simulink subsystem "AeroPropRefFranc"  (R2024b)
settings: Solver=VariableStepAuto  StartTime=0.0  StopTime=10.0  RelTol=1e-3
undefined symbols (not defined in the file or in its folder): ess, Force_b, Fprop_r, geom, H_b, Hdot_b, Moment_b, mot, mot2, mot3, mot4, Mprop_r, propel, propel2, propel3, propel4, pxf_diagram_options, SimIn, SimPar, tc, tc2, tc3, tc4
libraries: simulink x8, slpidlib x4, starslibAxisTransformations x2, libAxisTransformations x2
(part 8 of 10)

== system AeroPropRefFranc/Propulsion and Aerodynamic Forces and Moments/S-Function/Battery Model/powerplant/mot4/plant/mot4_plant_map_Pelec_funTW_volt_in/non-zero division ==
  note: original idea from Phil Sharer - ANL
      | original formula: u[1]\(u[2]+eps)*(u[2]!=0)
      | changes done by Gerald ZINI (dgey) - ANL (05\02\2001)
  note: (u[2]==0) is true then returns 1, thus (u[2]+(u[2]==0)) is equal to 0+1=1
  note: if u[2] == 0, then output == 0:
  note: (u[2]!=0) is false then returns 0
  note: and finally, the expression is: (u[1] \ 1) * 0 = 0
  note: (u[2]==0) is false then returns 0, thus (u[2]+(u[2]==0)) is equal to u[2]+0=u[2]
  note: if u[2] != 0, then output == u[1]\u[2]:
  note: (u[2]!=0) is true then returns 1
  note: and finally, the expression is: (u[1] \ u[2]) * 1 = u[1] \ u[2]
  In1 : Inport
  In2 : Inport  Port=2
  Fcn : Fcn  Expr=u[1]/(u[2]+(u[2]==0))*(u[2]!=0)
  Mux : Mux  Inputs=2
  Out1 : Outport
  wires:
  Mux/1 -> Fcn/1
  In1/1 -> Mux/1
  Fcn/1 -> Out1/1
  In2/1 -> Mux/2

== system AeroPropRefFranc/Propulsion and Aerodynamic Forces and Moments/S-Function/Battery Model/powerplant/propel/plant/propel_plant_uas/Propeller Power ==
  propel_plant_CT_simu : Inport
  propel_plant_CP_simu : Inport  Port=2
  propel_plant_thrust_simu : Inport  Port=3
  propel_plant_rps_simu : Inport  Port=4
  eqnmotion_plant_linvel_simu : Inport  Port=5
  Dot Product : DotProduct  OutDataTypeStr=Inherit: Inherit via internal rule
  Fcn : Fcn  Expr=u(2) / u(1) * u(4) * u(3) * propel.plant.init.propD
  Mux : Mux
  Product : Product
  Sqrt : Sqrt
  propel_plant_pwr_in_simu : Outport  VectorParamsAs1DForOutWhenUnconnected=off
  propel_plant_pwr_out_simu : Outport  Port=2  VectorParamsAs1DForOutWhenUnconnected=off
  wires:
  propel_plant_CP_simu/1 -> Mux/2
  Fcn/1 -> propel_plant_pwr_in_simu/1  "propel_plant_pwr_in_simu"
  propel_plant_rps_simu/1 -> Mux/4
  propel_plant_thrust_simu/1 -> Product/1, Mux/3
  propel_plant_CT_simu/1 -> Mux/1
  Mux/1 -> Fcn/1
  Product/1 -> propel_plant_pwr_out_simu/1
  Sqrt/1 -> Product/2  "tas"
  eqnmotion_plant_linvel_simu/1 -> Dot Product/2, Dot Product/1
  Dot Product/1 -> Sqrt/1

== system AeroPropRefFranc/Propulsion and Aerodynamic Forces and Moments/S-Function/Battery Model/powerplant/propel/plant/propel_plant_uas/Propeller_CP ==
  propel_plant_rps_simu : Inport
  propel_plant_init_CP_CT_map : Subsystem  mask{x=propel.plant.init.CP_CT_map(:,1)/60, map=propel.plant.init.CP_CT_map(:,3)}
  propel_plant_CP_simu : Outport  VectorParamsAs1DForOutWhenUnconnected=off
  wires:
  propel_plant_rps_simu/1 -> propel_plant_init_CP_CT_map/1(input x)
  propel_plant_init_CP_CT_map/1(output) -> propel_plant_CP_simu/1

== system AeroPropRefFranc/Propulsion and Aerodynamic Forces and Moments/S-Function/Battery Model/powerplant/propel/plant/propel_plant_uas/Propeller_Torque ==
  note: I = Wprop*R^2/3g
      | General Aviation Aircraft Design pg 619
  env_plant_density_simu : Inport
  propel_plant_CP_simu : Inport  Port=2
  tc_plant_trq_out_simu : Inport  Port=3
  tc_plant_inertia_out_simu : Inport  Port=4
  " " : Gain  Gain=-1
  "2pi " : Gain  Gain=1/2/pi
  Demux : Demux  Outputs=2
  Fcn1 : Fcn  Expr=(u(1)/(2*pi)) *u(3)*(u(2)^2)*(propel.plant.init.propD^5)
  Integrator1 : Integrator  InitialCondition=propel.ctrl.init.rps
  Mux : Mux  Inputs=3
  Product : Product  Inputs=*/
  Prop Inertia : Constant  Value=propel.plant.init.Iprop
  Sum1 : Sum  Inputs=|+-
  Sum2 : Sum  Inputs=|++
  Terminator : Terminator
  propel_plant_rps_simu : Outport  VectorParamsAs1DForOutWhenUnconnected=off
  propel_plant_restq_simu : Outport  Port=2  VectorParamsAs1DForOutWhenUnconnected=off
  wires:
  Product/1 -> "2pi "/1
  Sum1/1 -> Product/1
  Sum2/1 -> Product/2
  tc_plant_inertia_out_simu/1 -> Sum2/2
  Prop Inertia/1 -> Sum2/1
  Fcn1/1 -> " "/1, Sum1/2  "propel_plant_restq_simu"
  tc_plant_trq_out_simu/1 -> Demux/1
  propel_plant_CP_simu/1 -> Mux/1  "prop_plant_CP_simu"
  env_plant_density_simu/1 -> Mux/3  "env_plant_density_simu"
  Integrator1/1 -> Mux/2, propel_plant_rps_simu/1  "propeller_plant_rps_simu"
  " "/1 -> propel_plant_restq_simu/1
  Mux/1 -> Fcn1/1
  "2pi "/1 -> Integrator1/1
  Demux/1 -> Sum1/1
  Demux/2 -> Terminator/1

== system AeroPropRefFranc/Propulsion and Aerodynamic Forces and Moments/S-Function/Battery Model/powerplant/propel/plant/propel_plant_uas/Thrust_Generated ==
  env_plant_density_simu : Inport
  propel_plant_speed_simu : Inport  Port=2
  Mux5 : Mux  Inputs=3
  RPS2T : Fcn  Expr=u(2) * u(3) * propel.plant.init.propD^4 * u(1)^2
  propel_plant_init_CP_CT_map : Subsystem  mask{x=propel.plant.init.CP_CT_map(:,1)/60, map=propel.plant.init.CP_CT_map(:,2)}
  propel_plant_thrust_simu : Outport  VectorParamsAs1DForOutWhenUnconnected=off
  propel_plant_CT_simu : Outport  Port=2  VectorParamsAs1DForOutWhenUnconnected=off
  wires:
  RPS2T/1 -> propel_plant_thrust_simu/1
  Mux5/1 -> RPS2T/1
  propel_plant_speed_simu/1 -> Mux5/1, propel_plant_init_CP_CT_map/1(input x)
  env_plant_density_simu/1 -> Mux5/3
  propel_plant_init_CP_CT_map/1(output) -> Mux5/2, propel_plant_CT_simu/1

== system AeroPropRefFranc/Propulsion and Aerodynamic Forces and Moments/S-Function/Battery Model/powerplant/propel/plant/propel_plant_uas/Total_Moment ==
  propel_plant_thrust_simu : Inport
  propel_plant_restq_simu : Inport  Port=2
  Gain : Gain  Gain=-propel.plant.init.rotationdir
  Gain1 : Gain  Gain=propel.plant.init.thrustdir
  Moment_due_to_eng_position : Subsystem
  Sum2 : Sum  Inputs=|+-  SaturateOnIntegerOverflow=on
  Sum4 : Sum  SaturateOnIntegerOverflow=on
  geom.init.CG : Constant  Value=geom.init.CG
  propel.plant.init.pos : Constant  Value=propel.plant.init.pos
  accmoment_plant_totmoment_simu : Outport  VectorParamsAs1DForOutWhenUnconnected=off
  wires:
  Moment_due_to_eng_position/1(X Prod) -> Sum4/1
  propel_plant_thrust_simu/1 -> Gain1/1
  geom.init.CG/1 -> Sum2/2
  propel.plant.init.pos/1 -> Sum2/1
  Sum4/1 -> accmoment_plant_totmoment_simu/1  "accmoment_plant_totmoment_simu"
  Sum2/1 -> Moment_due_to_eng_position/1(Vec 1)
  Gain/1 -> Sum4/2
  Gain1/1 -> Moment_due_to_eng_position/2(Vec 2)
  propel_plant_restq_simu/1 -> Gain/1

== system AeroPropRefFranc/Propulsion and Aerodynamic Forces and Moments/S-Function/Battery Model/powerplant/propel2/plant/propel2_plant_uas/Propeller Power ==
  propel_plant_CT_simu : Inport
  propel_plant_CP_simu : Inport  Port=2
  propel_plant_thrust_simu : Inport  Port=3
  propel_plant_rps_simu : Inport  Port=4
  eqnmotion_plant_linvel_simu : Inport  Port=5
  Dot Product : DotProduct  OutDataTypeStr=Inherit: Inherit via internal rule
  Fcn : Fcn  Expr=u(2) / u(1) * u(4) * u(3) * propel2.plant.init.propD
  Mux : Mux
  Product : Product
  Sqrt : Sqrt
  propel_plant_pwr_in_simu : Outport  VectorParamsAs1DForOutWhenUnconnected=off
  propel_plant_pwr_out_simu : Outport  Port=2  VectorParamsAs1DForOutWhenUnconnected=off
  wires:
  propel_plant_CP_simu/1 -> Mux/2
  Fcn/1 -> propel_plant_pwr_in_simu/1  "propel_plant_pwr_in_simu"
  propel_plant_rps_simu/1 -> Mux/4
  propel_plant_thrust_simu/1 -> Product/1, Mux/3
  propel_plant_CT_simu/1 -> Mux/1
  Mux/1 -> Fcn/1
  Product/1 -> propel_plant_pwr_out_simu/1
  Sqrt/1 -> Product/2  "tas"
  eqnmotion_plant_linvel_simu/1 -> Dot Product/2, Dot Product/1
  Dot Product/1 -> Sqrt/1

== system AeroPropRefFranc/Propulsion and Aerodynamic Forces and Moments/S-Function/Battery Model/powerplant/propel2/plant/propel2_plant_uas/Propeller_CP ==
  propel_plant_rps_simu : Inport
  propel_plant_init_CP_CT_map : Subsystem  mask{x=propel2.plant.init.CP_CT_map(:,1)/60, map=propel2.plant.init.CP_CT_map(:,3)}
  propel_plant_CP_simu : Outport  VectorParamsAs1DForOutWhenUnconnected=off
  wires:
  propel_plant_rps_simu/1 -> propel_plant_init_CP_CT_map/1(input x)
  propel_plant_init_CP_CT_map/1(output) -> propel_plant_CP_simu/1

== system AeroPropRefFranc/Propulsion and Aerodynamic Forces and Moments/S-Function/Battery Model/powerplant/propel2/plant/propel2_plant_uas/Propeller_Torque ==
  note: I = Wprop*R^2/3g
      | General Aviation Aircraft Design pg 619
  env_plant_density_simu : Inport
  propel_plant_CP_simu : Inport  Port=2
  tc_plant_trq_out_simu : Inport  Port=3
  tc_plant_inertia_out_simu : Inport  Port=4
  " " : Gain  Gain=-1
  "2pi " : Gain  Gain=1/2/pi
  Demux : Demux  Outputs=2
  Fcn1 : Fcn  Expr=(u(1)/(2*pi)) *u(3)*(u(2)^2)*(propel2.plant.init.propD^5)
  Integrator1 : Integrator  InitialCondition=propel2.ctrl.init.rps
  Mux : Mux  Inputs=3
  Product : Product  Inputs=*/
  Prop Inertia : Constant  Value=propel2.plant.init.Iprop
  Sum1 : Sum  Inputs=|+-
  Sum2 : Sum  Inputs=|++
  Terminator : Terminator
  propel_plant_rps_simu : Outport  VectorParamsAs1DForOutWhenUnconnected=off
  propel_plant_restq_simu : Outport  Port=2  VectorParamsAs1DForOutWhenUnconnected=off
  wires:
  Product/1 -> "2pi "/1
  Sum1/1 -> Product/1
  Sum2/1 -> Product/2
  tc_plant_inertia_out_simu/1 -> Sum2/2
  Prop Inertia/1 -> Sum2/1
  Fcn1/1 -> " "/1, Sum1/2  "propel_plant_restq_simu"
  tc_plant_trq_out_simu/1 -> Demux/1
  propel_plant_CP_simu/1 -> Mux/1  "prop_plant_CP_simu"
  env_plant_density_simu/1 -> Mux/3  "env_plant_density_simu"
  Integrator1/1 -> Mux/2, propel_plant_rps_simu/1  "propeller_plant_rps_simu"
  " "/1 -> propel_plant_restq_simu/1
  Mux/1 -> Fcn1/1
  "2pi "/1 -> Integrator1/1
  Demux/1 -> Sum1/1
  Demux/2 -> Terminator/1

== system AeroPropRefFranc/Propulsion and Aerodynamic Forces and Moments/S-Function/Battery Model/powerplant/propel2/plant/propel2_plant_uas/Thrust_Generated ==
  env_plant_density_simu : Inport
  propel_plant_speed_simu : Inport  Port=2
  Mux5 : Mux  Inputs=3
  RPS2T : Fcn  Expr=u(2) * u(3) * propel2.plant.init.propD^4 * u(1)^2
  propel_plant_init_CP_CT_map : Subsystem  mask{x=propel2.plant.init.CP_CT_map(:,1)/60, map=propel2.plant.init.CP_CT_map(:,2)}
  propel_plant_thrust_simu : Outport  VectorParamsAs1DForOutWhenUnconnected=off
  propel_plant_CT_simu : Outport  Port=2  VectorParamsAs1DForOutWhenUnconnected=off
  wires:
  RPS2T/1 -> propel_plant_thrust_simu/1
  Mux5/1 -> RPS2T/1
  propel_plant_speed_simu/1 -> Mux5/1, propel_plant_init_CP_CT_map/1(input x)
  env_plant_density_simu/1 -> Mux5/3
  propel_plant_init_CP_CT_map/1(output) -> Mux5/2, propel_plant_CT_simu/1

== system AeroPropRefFranc/Propulsion and Aerodynamic Forces and Moments/S-Function/Battery Model/powerplant/propel2/plant/propel2_plant_uas/Total_Moment ==
  propel_plant_thrust_simu : Inport
  propel_plant_restq_simu : Inport  Port=2
  Gain : Gain  Gain=-propel2.plant.init.rotationdir
  Gain1 : Gain  Gain=propel2.plant.init.thrustdir
  Moment_due_to_eng_position : Subsystem
  Sum2 : Sum  Inputs=|+-  SaturateOnIntegerOverflow=on
  Sum4 : Sum  SaturateOnIntegerOverflow=on
  geom.init.CG : Constant  Value=geom.init.CG
  propel.plant.init.pos : Constant  Value=propel2.plant.init.pos
  accmoment_plant_totmoment_simu : Outport  VectorParamsAs1DForOutWhenUnconnected=off
  wires:
  Moment_due_to_eng_position/1(X Prod) -> Sum4/1
  propel_plant_thrust_simu/1 -> Gain1/1
  geom.init.CG/1 -> Sum2/2
  propel.plant.init.pos/1 -> Sum2/1
  Sum4/1 -> accmoment_plant_totmoment_simu/1  "accmoment_plant_totmoment_simu"
  Sum2/1 -> Moment_due_to_eng_position/1(Vec 1)
  Gain/1 -> Sum4/2
  Gain1/1 -> Moment_due_to_eng_position/2(Vec 2)
  propel_plant_restq_simu/1 -> Gain/1

== system AeroPropRefFranc/Propulsion and Aerodynamic Forces and Moments/S-Function/Battery Model/powerplant/propel3/plant/propel3_plant_uas/Propeller Power ==
  propel_plant_CT_simu : Inport
  propel_plant_CP_simu : Inport  Port=2
  propel_plant_thrust_simu : Inport  Port=3
  propel_plant_rps_simu : Inport  Port=4
  eqnmotion_plant_linvel_simu : Inport  Port=5
  Dot Product : DotProduct  OutDataTypeStr=Inherit: Inherit via internal rule
  Fcn : Fcn  Expr=u(2) / u(1) * u(4) * u(3) * propel3.plant.init.propD
  Mux : Mux
  Product : Product
  Sqrt : Sqrt
  propel_plant_pwr_in_simu : Outport  VectorParamsAs1DForOutWhenUnconnected=off
  propel_plant_pwr_out_simu : Outport  Port=2  VectorParamsAs1DForOutWhenUnconnected=off
  wires:
  propel_plant_CP_simu/1 -> Mux/2
  Fcn/1 -> propel_plant_pwr_in_simu/1  "propel_plant_pwr_in_simu"
  propel_plant_rps_simu/1 -> Mux/4
  propel_plant_thrust_simu/1 -> Product/1, Mux/3
  propel_plant_CT_simu/1 -> Mux/1
  Mux/1 -> Fcn/1
  Product/1 -> propel_plant_pwr_out_simu/1
  Sqrt/1 -> Product/2  "tas"
  eqnmotion_plant_linvel_simu/1 -> Dot Product/2, Dot Product/1
  Dot Product/1 -> Sqrt/1

== system AeroPropRefFranc/Propulsion and Aerodynamic Forces and Moments/S-Function/Battery Model/powerplant/propel3/plant/propel3_plant_uas/Propeller_CP ==
  propel_plant_rps_simu : Inport
  propel_plant_init_CP_CT_map : Subsystem  mask{x=propel3.plant.init.CP_CT_map(:,1)/60, map=propel3.plant.init.CP_CT_map(:,3)}
  propel_plant_CP_simu : Outport  VectorParamsAs1DForOutWhenUnconnected=off
  wires:
  propel_plant_rps_simu/1 -> propel_plant_init_CP_CT_map/1(input x)
  propel_plant_init_CP_CT_map/1(output) -> propel_plant_CP_simu/1

== system AeroPropRefFranc/Propulsion and Aerodynamic Forces and Moments/S-Function/Battery Model/powerplant/propel3/plant/propel3_plant_uas/Propeller_Torque ==
  note: I = Wprop*R^2/3g
      | General Aviation Aircraft Design pg 619
  env_plant_density_simu : Inport
  propel_plant_CP_simu : Inport  Port=2
  tc_plant_trq_out_simu : Inport  Port=3
  tc_plant_inertia_out_simu : Inport  Port=4
  " " : Gain  Gain=-1
  "2pi " : Gain  Gain=1/2/pi
  Demux : Demux  Outputs=2
  Fcn1 : Fcn  Expr=(u(1)/(2*pi)) *u(3)*(u(2)^2)*(propel3.plant.init.propD^5)
  Integrator1 : Integrator  InitialCondition=propel3.ctrl.init.rps
  Mux : Mux  Inputs=3
  Product : Product  Inputs=*/
  Prop Inertia : Constant  Value=propel3.plant.init.Iprop
  Sum1 : Sum  Inputs=|+-
  Sum2 : Sum  Inputs=|++
  Terminator : Terminator
  propel_plant_rps_simu : Outport  VectorParamsAs1DForOutWhenUnconnected=off
  propel_plant_restq_simu : Outport  Port=2  VectorParamsAs1DForOutWhenUnconnected=off
  wires:
  Product/1 -> "2pi "/1
  Sum1/1 -> Product/1
  Sum2/1 -> Product/2
  tc_plant_inertia_out_simu/1 -> Sum2/2
  Prop Inertia/1 -> Sum2/1
  Fcn1/1 -> " "/1, Sum1/2  "propel_plant_restq_simu"
  tc_plant_trq_out_simu/1 -> Demux/1
  propel_plant_CP_simu/1 -> Mux/1  "prop_plant_CP_simu"
  env_plant_density_simu/1 -> Mux/3  "env_plant_density_simu"
  Integrator1/1 -> Mux/2, propel_plant_rps_simu/1  "propeller_plant_rps_simu"
  " "/1 -> propel_plant_restq_simu/1
  Mux/1 -> Fcn1/1
  "2pi "/1 -> Integrator1/1
  Demux/1 -> Sum1/1
  Demux/2 -> Terminator/1

== system AeroPropRefFranc/Propulsion and Aerodynamic Forces and Moments/S-Function/Battery Model/powerplant/propel3/plant/propel3_plant_uas/Thrust_Generated ==
  env_plant_density_simu : Inport
  propel_plant_speed_simu : Inport  Port=2
  Mux5 : Mux  Inputs=3
  RPS2T : Fcn  Expr=u(2) * u(3) * propel3.plant.init.propD^4 * u(1)^2
  propel_plant_init_CP_CT_map : Subsystem  mask{x=propel3.plant.init.CP_CT_map(:,1)/60, map=propel3.plant.init.CP_CT_map(:,2)}
  propel_plant_thrust_simu : Outport  VectorParamsAs1DForOutWhenUnconnected=off
  propel_plant_CT_simu : Outport  Port=2  VectorParamsAs1DForOutWhenUnconnected=off
  wires:
  RPS2T/1 -> propel_plant_thrust_simu/1
  Mux5/1 -> RPS2T/1
  propel_plant_speed_simu/1 -> Mux5/1, propel_plant_init_CP_CT_map/1(input x)
  env_plant_density_simu/1 -> Mux5/3
  propel_plant_init_CP_CT_map/1(output) -> Mux5/2, propel_plant_CT_simu/1

== system AeroPropRefFranc/Propulsion and Aerodynamic Forces and Moments/S-Function/Battery Model/powerplant/propel3/plant/propel3_plant_uas/Total_Moment ==
  propel_plant_thrust_simu : Inport
  propel_plant_restq_simu : Inport  Port=2
  Gain : Gain  Gain=-propel3.plant.init.rotationdir
  Gain1 : Gain  Gain=propel3.plant.init.thrustdir
  Moment_due_to_eng_position : Subsystem
  Sum2 : Sum  Inputs=|+-  SaturateOnIntegerOverflow=on
  Sum4 : Sum  SaturateOnIntegerOverflow=on
  geom.init.CG : Constant  Value=geom.init.CG
  propel.plant.init.pos : Constant  Value=propel3.plant.init.pos
  accmoment_plant_totmoment_simu : Outport  VectorParamsAs1DForOutWhenUnconnected=off
  wires:
  Moment_due_to_eng_position/1(X Prod) -> Sum4/1
  propel_plant_thrust_simu/1 -> Gain1/1
  geom.init.CG/1 -> Sum2/2
  propel.plant.init.pos/1 -> Sum2/1
  Sum4/1 -> accmoment_plant_totmoment_simu/1  "accmoment_plant_totmoment_simu"
  Sum2/1 -> Moment_due_to_eng_position/1(Vec 1)
  Gain/1 -> Sum4/2
  Gain1/1 -> Moment_due_to_eng_position/2(Vec 2)
  propel_plant_restq_simu/1 -> Gain/1

== system AeroPropRefFranc/Propulsion and Aerodynamic Forces and Moments/S-Function/Battery Model/powerplant/propel4/plant/propel4_plant_uas/Propeller Power ==
  propel_plant_CT_simu : Inport
  propel_plant_CP_simu : Inport  Port=2
  propel_plant_thrust_simu : Inport  Port=3
  propel_plant_rps_simu : Inport  Port=4
  eqnmotion_plant_linvel_simu : Inport  Port=5
  Dot Product : DotProduct  OutDataTypeStr=Inherit: Inherit via internal rule
  Fcn : Fcn  Expr=u(2) / u(1) * u(4) * u(3) * propel4.plant.init.propD
  Mux : Mux
  Product : Product
  Sqrt : Sqrt
  propel_plant_pwr_in_simu : Outport  VectorParamsAs1DForOutWhenUnconnected=off
  propel_plant_pwr_out_simu : Outport  Port=2  VectorParamsAs1DForOutWhenUnconnected=off
  wires:
  propel_plant_CP_simu/1 -> Mux/2
  Fcn/1 -> propel_plant_pwr_in_simu/1  "propel_plant_pwr_in_simu"
  propel_plant_rps_simu/1 -> Mux/4
  propel_plant_thrust_simu/1 -> Product/1, Mux/3
  propel_plant_CT_simu/1 -> Mux/1
  Mux/1 -> Fcn/1
  Product/1 -> propel_plant_pwr_out_simu/1
  Sqrt/1 -> Product/2  "tas"
  eqnmotion_plant_linvel_simu/1 -> Dot Product/2, Dot Product/1
  Dot Product/1 -> Sqrt/1

== system AeroPropRefFranc/Propulsion and Aerodynamic Forces and Moments/S-Function/Battery Model/powerplant/propel4/plant/propel4_plant_uas/Propeller_CP ==
  propel_plant_rps_simu : Inport
  propel_plant_init_CP_CT_map : Subsystem  mask{x=propel4.plant.init.CP_CT_map(:,1)/60, map=propel4.plant.init.CP_CT_map(:,3)}
  propel_plant_CP_simu : Outport  VectorParamsAs1DForOutWhenUnconnected=off
  wires:
  propel_plant_rps_simu/1 -> propel_plant_init_CP_CT_map/1(input x)
  propel_plant_init_CP_CT_map/1(output) -> propel_plant_CP_simu/1

== system AeroPropRefFranc/Propulsion and Aerodynamic Forces and Moments/S-Function/Battery Model/powerplant/propel4/plant/propel4_plant_uas/Propeller_Torque ==
  note: I = Wprop*R^2/3g
      | General Aviation Aircraft Design pg 619
  env_plant_density_simu : Inport
  propel_plant_CP_simu : Inport  Port=2
  tc_plant_trq_out_simu : Inport  Port=3
  tc_plant_inertia_out_simu : Inport  Port=4
  " " : Gain  Gain=-1
  "2pi " : Gain  Gain=1/2/pi
  Demux : Demux  Outputs=2
  Fcn1 : Fcn  Expr=(u(1)/(2*pi)) *u(3)*(u(2)^2)*(propel4.plant.init.propD^5)
  Integrator1 : Integrator  InitialCondition=propel4.ctrl.init.rps
  Mux : Mux  Inputs=3
  Product : Product  Inputs=*/
  Prop Inertia : Constant  Value=propel4.plant.init.Iprop
  Sum1 : Sum  Inputs=|+-
  Sum2 : Sum  Inputs=|++
  Terminator : Terminator
  propel_plant_rps_simu : Outport  VectorParamsAs1DForOutWhenUnconnected=off
  propel_plant_restq_simu : Outport  Port=2  VectorParamsAs1DForOutWhenUnconnected=off
  wires:
  Product/1 -> "2pi "/1
  Sum1/1 -> Product/1
  Sum2/1 -> Product/2
  tc_plant_inertia_out_simu/1 -> Sum2/2
  Prop Inertia/1 -> Sum2/1
  Fcn1/1 -> " "/1, Sum1/2  "propel_plant_restq_simu"
  tc_plant_trq_out_simu/1 -> Demux/1
  propel_plant_CP_simu/1 -> Mux/1  "prop_plant_CP_simu"
  env_plant_density_simu/1 -> Mux/3  "env_plant_density_simu"
  Integrator1/1 -> Mux/2, propel_plant_rps_simu/1  "propeller_plant_rps_simu"
  " "/1 -> propel_plant_restq_simu/1
  Mux/1 -> Fcn1/1
  "2pi "/1 -> Integrator1/1
  Demux/1 -> Sum1/1
  Demux/2 -> Terminator/1

== system AeroPropRefFranc/Propulsion and Aerodynamic Forces and Moments/S-Function/Battery Model/powerplant/propel4/plant/propel4_plant_uas/Thrust_Generated ==
  env_plant_density_simu : Inport
  propel_plant_speed_simu : Inport  Port=2
  Mux5 : Mux  Inputs=3
  RPS2T : Fcn  Expr=u(2) * u(3) * propel4.plant.init.propD^4 * u(1)^2
  propel_plant_init_CP_CT_map : Subsystem  mask{x=propel4.plant.init.CP_CT_map(:,1)/60, map=propel4.plant.init.CP_CT_map(:,2)}
  propel_plant_thrust_simu : Outport  VectorParamsAs1DForOutWhenUnconnected=off
  propel_plant_CT_simu : Outport  Port=2  VectorParamsAs1DForOutWhenUnconnected=off
  wires:
  RPS2T/1 -> propel_plant_thrust_simu/1
  Mux5/1 -> RPS2T/1
  propel_plant_speed_simu/1 -> Mux5/1, propel_plant_init_CP_CT_map/1(input x)
  env_plant_density_simu/1 -> Mux5/3
  propel_plant_init_CP_CT_map/1(output) -> Mux5/2, propel_plant_CT_simu/1

== system AeroPropRefFranc/Propulsion and Aerodynamic Forces and Moments/S-Function/Battery Model/powerplant/propel4/plant/propel4_plant_uas/Total_Moment ==
  propel_plant_thrust_simu : Inport
  propel_plant_restq_simu : Inport  Port=2
  Gain : Gain  Gain=-propel4.plant.init.rotationdir
  Gain1 : Gain  Gain=propel4.plant.init.thrustdir
  Moment_due_to_eng_position : Subsystem
  Sum2 : Sum  Inputs=|+-  SaturateOnIntegerOverflow=on
  Sum4 : Sum  SaturateOnIntegerOverflow=on
  geom.init.CG : Constant  Value=geom.init.CG
  propel.plant.init.pos : Constant  Value=propel4.plant.init.pos
  accmoment_plant_totmoment_simu : Outport  VectorParamsAs1DForOutWhenUnconnected=off
  wires:
  Moment_due_to_eng_position/1(X Prod) -> Sum4/1
  propel_plant_thrust_simu/1 -> Gain1/1
  geom.init.CG/1 -> Sum2/2
  propel.plant.init.pos/1 -> Sum2/1
  Sum4/1 -> accmoment_plant_totmoment_simu/1  "accmoment_plant_totmoment_simu"
  Sum2/1 -> Moment_due_to_eng_position/1(Vec 1)
  Gain/1 -> Sum4/2
  Gain1/1 -> Moment_due_to_eng_position/2(Vec 2)
  propel_plant_restq_simu/1 -> Gain/1

== system AeroPropRefFranc/Propulsion and Aerodynamic Forces and Moments/S-Function/Battery Model/powerplant/tc/plant/tc_plant_map_trqloss_funTW/Inertia calculation ==
  inertia in : Inport
  Sum3 : Sum  Inputs=|++  InputSameDT=on  SaturateOnIntegerOverflow=on  OutDataTypeStr=Inherit: Same as first input
  tc inertia : Constant  Value=tc.plant.init.inertia
  tc.plant.init.ratio : Gain  Gain=tc.plant.init.ratio
  "tc.plant.init.ratio " : Gain  Gain=tc.plant.init.ratio
  inertia out : Outport
  wires:
  Sum3/1 -> inertia out/1
  tc inertia/1 -> Sum3/2
  tc.plant.init.ratio/1 -> Sum3/1
  inertia in/1 -> "tc.plant.init.ratio "/1
  "tc.plant.init.ratio "/1 -> tc.plant.init.ratio/1

== system AeroPropRefFranc/Propulsion and Aerodynamic Forces and Moments/S-Function/Battery Model/powerplant/tc/plant/tc_plant_map_trqloss_funTW/Speed calculation ==
  spd out : Inport
  tc.plant.init.ratio : Gain  Gain=tc.plant.init.ratio
  spd in : Outport
  wires:
  tc.plant.init.ratio/1 -> spd in/1
  spd out/1 -> tc.plant.init.ratio/1

== system AeroPropRefFranc/Propulsion and Aerodynamic Forces and Moments/S-Function/Battery Model/powerplant/tc/plant/tc_plant_map_trqloss_funTW/Torque calculation ==
  spd in : Inport
  trq in : Inport  Port=2
  Abs : Abs
  Abs1 : Abs
  Blending (state dependent) : Subsystem  mask(State dependent blending){xl=-tc.plant.init.spd_thresh, yl=-1, xc=0, yc=0, xr=tc.plant.init.spd_thresh, yr=1}
      mask prompts: xl "Left point (x):"; yl "Left point (y):"; xc "Center point (x):"; yc "Center point (y):"; xr "Right point (x):"; yr "Right point (y):"
      mask help: This block implements state dependent smoothing/blending. IMPORTANT: See help menu.
      mask Help: The output equals the product of the first input and a "hat" function defined by the three points specified in the dialog box.  The second input forms the argument to the hat function.\n\nIMPORTANT: A divide by zero error will result if first coordinates of the three points specified for the hat function are NOT distinct.
      mask Display: plot([-1 1 3 6 8], [1.5 1.5 0.5 4.0 4.0])
  Sum2 : Sum  Inputs=|+-  InputSameDT=on  SaturateOnIntegerOverflow=on  OutDataTypeStr=Inherit: Same as first input
  tc.plant.init.ratio : Gain  Gain=tc.plant.init.ratio
  trq losses : Subsystem  mask(Lookup Table (2-D)){x=tc.plant.init.trq_loss.idx1_trq, y=tc.plant.init.trq_loss.idx2_spd, t=tc.plant.init.trq_loss.map}
      mask prompts: x "Row:"; y "Column:"; t "Table:"
      mask help: Performs 2-D linear interpolation of input values using the specified input/output table. Extrapolation is performed outside the table boundaries.
      mask init:
      | [r,c]=size(t);
      | xt=reshape(x,prod(size(x)),1);
      | xi=xt(:,ones(1,c));
      | minx=min(x); maxx=max(x);
      | mint=min(min(t)); maxt=max(max(t));
      mask Display: plot(xi,t,[minx maxx],[mint mint],[minx minx],[mint maxt])
  trq out : Outport
  wires:
  Abs/1 -> trq losses/1(Rows)
  Abs1/1 -> trq losses/2(Cols)
  trq losses/1(Out1) -> Blending (state dependent)/1(Input)
  Blending (state dependent)/1(Output) -> Sum2/2
  spd in/1 -> Abs1/1, Blending (state dependent)/2(Control (state))
  trq in/1 -> Abs/1, Sum2/1
  Sum2/1 -> tc.plant.init.ratio/1
  tc.plant.init.ratio/1 -> trq out/1

== system AeroPropRefFranc/Propulsion and Aerodynamic Forces and Moments/S-Function/Battery Model/powerplant/tc2/plant/tc2_plant_map_trqloss_funTW/Inertia calculation ==
  inertia in : Inport
  Sum3 : Sum  Inputs=|++  InputSameDT=on  SaturateOnIntegerOverflow=on  OutDataTypeStr=Inherit: Same as first input
  tc inertia : Constant  Value=tc2.plant.init.inertia
  tc.plant.init.ratio : Gain  Gain=tc2.plant.init.ratio
  "tc.plant.init.ratio " : Gain  Gain=tc2.plant.init.ratio
  inertia out : Outport
  wires:
  Sum3/1 -> inertia out/1
  tc inertia/1 -> Sum3/2
  tc.plant.init.ratio/1 -> Sum3/1
  inertia in/1 -> "tc.plant.init.ratio "/1
  "tc.plant.init.ratio "/1 -> tc.plant.init.ratio/1

== system AeroPropRefFranc/Propulsion and Aerodynamic Forces and Moments/S-Function/Battery Model/powerplant/tc2/plant/tc2_plant_map_trqloss_funTW/Speed calculation ==
  spd out : Inport
  tc.plant.init.ratio : Gain  Gain=tc2.plant.init.ratio
  spd in : Outport
  wires:
  tc.plant.init.ratio/1 -> spd in/1
  spd out/1 -> tc.plant.init.ratio/1

== system AeroPropRefFranc/Propulsion and Aerodynamic Forces and Moments/S-Function/Battery Model/powerplant/tc2/plant/tc2_plant_map_trqloss_funTW/Torque calculation ==
  spd in : Inport
  trq in : Inport  Port=2
  Abs : Abs
  Abs1 : Abs
  Blending (state dependent) : Subsystem  mask(State dependent blending){xl=-tc2.plant.init.spd_thresh, yl=-1, xc=0, yc=0, xr=tc2.plant.init.spd_thresh, yr=1}
      mask prompts: xl "Left point (x):"; yl "Left point (y):"; xc "Center point (x):"; yc "Center point (y):"; xr "Right point (x):"; yr "Right point (y):"
      mask help: This block implements state dependent smoothing/blending. IMPORTANT: See help menu.
      mask Help: The output equals the product of the first input and a "hat" function defined by the three points specified in the dialog box.  The second input forms the argument to the hat function.\n\nIMPORTANT: A divide by zero error will result if first coordinates of the three points specified for the hat function are NOT distinct.
      mask Display: plot([-1 1 3 6 8], [1.5 1.5 0.5 4.0 4.0])
  Sum2 : Sum  Inputs=|+-  InputSameDT=on  SaturateOnIntegerOverflow=on  OutDataTypeStr=Inherit: Same as first input
  tc.plant.init.ratio : Gain  Gain=tc2.plant.init.ratio
  trq losses : Subsystem  mask(Lookup Table (2-D)){x=tc2.plant.init.trq_loss.idx1_trq, y=tc2.plant.init.trq_loss.idx2_spd, t=tc2.plant.init.trq_loss.map}
      mask prompts: x "Row:"; y "Column:"; t "Table:"
      mask help: Performs 2-D linear interpolation of input values using the specified input/output table. Extrapolation is performed outside the table boundaries.
      mask init:
      | [r,c]=size(t);
      | xt=reshape(x,prod(size(x)),1);
      | xi=xt(:,ones(1,c));
      | minx=min(x); maxx=max(x);
      | mint=min(min(t)); maxt=max(max(t));
      mask Display: plot(xi,t,[minx maxx],[mint mint],[minx minx],[mint maxt])
  trq out : Outport
  wires:
  Abs/1 -> trq losses/1(Rows)
  Abs1/1 -> trq losses/2(Cols)
  trq losses/1(Out1) -> Blending (state dependent)/1(Input)
  Blending (state dependent)/1(Output) -> Sum2/2
  spd in/1 -> Abs1/1, Blending (state dependent)/2(Control (state))
  trq in/1 -> Abs/1, Sum2/1
  Sum2/1 -> tc.plant.init.ratio/1
  tc.plant.init.ratio/1 -> trq out/1

== system AeroPropRefFranc/Propulsion and Aerodynamic Forces and Moments/S-Function/Battery Model/powerplant/tc3/plant/tc3_plant_map_trqloss_funTW/Inertia calculation ==
  inertia in : Inport
  Sum3 : Sum  Inputs=|++  InputSameDT=on  SaturateOnIntegerOverflow=on  OutDataTypeStr=Inherit: Same as first input
  tc inertia : Constant  Value=tc3.plant.init.inertia
  tc.plant.init.ratio : Gain  Gain=tc3.plant.init.ratio
  "tc.plant.init.ratio " : Gain  Gain=tc3.plant.init.ratio
  inertia out : Outport
  wires:
  Sum3/1 -> inertia out/1
  tc inertia/1 -> Sum3/2
  tc.plant.init.ratio/1 -> Sum3/1
  inertia in/1 -> "tc.plant.init.ratio "/1
  "tc.plant.init.ratio "/1 -> tc.plant.init.ratio/1

== system AeroPropRefFranc/Propulsion and Aerodynamic Forces and Moments/S-Function/Battery Model/powerplant/tc3/plant/tc3_plant_map_trqloss_funTW/Speed calculation ==
  spd out : Inport
  tc.plant.init.ratio : Gain  Gain=tc3.plant.init.ratio
  spd in : Outport
  wires:
  tc.plant.init.ratio/1 -> spd in/1
  spd out/1 -> tc.plant.init.ratio/1

== system AeroPropRefFranc/Propulsion and Aerodynamic Forces and Moments/S-Function/Battery Model/powerplant/tc3/plant/tc3_plant_map_trqloss_funTW/Torque calculation ==
  spd in : Inport
  trq in : Inport  Port=2
  Abs : Abs
  Abs1 : Abs
  Blending (state dependent) : Subsystem  mask(State dependent blending){xl=-tc3.plant.init.spd_thresh, yl=-1, xc=0, yc=0, xr=tc3.plant.init.spd_thresh, yr=1}
      mask prompts: xl "Left point (x):"; yl "Left point (y):"; xc "Center point (x):"; yc "Center point (y):"; xr "Right point (x):"; yr "Right point (y):"
      mask help: This block implements state dependent smoothing/blending. IMPORTANT: See help menu.
      mask Help: The output equals the product of the first input and a "hat" function defined by the three points specified in the dialog box.  The second input forms the argument to the hat function.\n\nIMPORTANT: A divide by zero error will result if first coordinates of the three points specified for the hat function are NOT distinct.
      mask Display: plot([-1 1 3 6 8], [1.5 1.5 0.5 4.0 4.0])
  Sum2 : Sum  Inputs=|+-  InputSameDT=on  SaturateOnIntegerOverflow=on  OutDataTypeStr=Inherit: Same as first input
  tc.plant.init.ratio : Gain  Gain=tc3.plant.init.ratio
  trq losses : Subsystem  mask(Lookup Table (2-D)){x=tc3.plant.init.trq_loss.idx1_trq, y=tc3.plant.init.trq_loss.idx2_spd, t=tc3.plant.init.trq_loss.map}
      mask prompts: x "Row:"; y "Column:"; t "Table:"
      mask help: Performs 2-D linear interpolation of input values using the specified input/output table. Extrapolation is performed outside the table boundaries.
      mask init:
      | [r,c]=size(t);
      | xt=reshape(x,prod(size(x)),1);
      | xi=xt(:,ones(1,c));
      | minx=min(x); maxx=max(x);
      | mint=min(min(t)); maxt=max(max(t));
      mask Display: plot(xi,t,[minx maxx],[mint mint],[minx minx],[mint maxt])
  trq out : Outport
  wires:
  Abs/1 -> trq losses/1(Rows)
  Abs1/1 -> trq losses/2(Cols)
  trq losses/1(Out1) -> Blending (state dependent)/1(Input)
  Blending (state dependent)/1(Output) -> Sum2/2
  spd in/1 -> Abs1/1, Blending (state dependent)/2(Control (state))
  trq in/1 -> Abs/1, Sum2/1
  Sum2/1 -> tc.plant.init.ratio/1
  tc.plant.init.ratio/1 -> trq out/1

== system AeroPropRefFranc/Propulsion and Aerodynamic Forces and Moments/S-Function/Battery Model/powerplant/tc4/plant/tc4_plant_map_trqloss_funTW/Inertia calculation ==
  inertia in : Inport
  Sum3 : Sum  Inputs=|++  InputSameDT=on  SaturateOnIntegerOverflow=on  OutDataTypeStr=Inherit: Same as first input
  tc inertia : Constant  Value=tc4.plant.init.inertia
  tc.plant.init.ratio : Gain  Gain=tc4.plant.init.ratio
  "tc.plant.init.ratio " : Gain  Gain=tc4.plant.init.ratio
  inertia out : Outport
  wires:
  Sum3/1 -> inertia out/1
  tc inertia/1 -> Sum3/2
  tc.plant.init.ratio/1 -> Sum3/1
  inertia in/1 -> "tc.plant.init.ratio "/1
  "tc.plant.init.ratio "/1 -> tc.plant.init.ratio/1

== system AeroPropRefFranc/Propulsion and Aerodynamic Forces and Moments/S-Function/Battery Model/powerplant/tc4/plant/tc4_plant_map_trqloss_funTW/Speed calculation ==
  spd out : Inport
  tc.plant.init.ratio : Gain  Gain=tc4.plant.init.ratio
  spd in : Outport
  wires:
  tc.plant.init.ratio/1 -> spd in/1
  spd out/1 -> tc.plant.init.ratio/1

== system AeroPropRefFranc/Propulsion and Aerodynamic Forces and Moments/S-Function/Battery Model/powerplant/tc4/plant/tc4_plant_map_trqloss_funTW/Torque calculation ==
  spd in : Inport
  trq in : Inport  Port=2
  Abs : Abs
  Abs1 : Abs
  Blending (state dependent) : Subsystem  mask(State dependent blending){xl=-tc4.plant.init.spd_thresh, yl=-1, xc=0, yc=0, xr=tc4.plant.init.spd_thresh, yr=1}
      mask prompts: xl "Left point (x):"; yl "Left point (y):"; xc "Center point (x):"; yc "Center point (y):"; xr "Right point (x):"; yr "Right point (y):"
      mask help: This block implements state dependent smoothing/blending. IMPORTANT: See help menu.
      mask Help: The output equals the product of the first input and a "hat" function defined by the three points specified in the dialog box.  The second input forms the argument to the hat function.\n\nIMPORTANT: A divide by zero error will result if first coordinates of the three points specified for the hat function are NOT distinct.
      mask Display: plot([-1 1 3 6 8], [1.5 1.5 0.5 4.0 4.0])
  Sum2 : Sum  Inputs=|+-  InputSameDT=on  SaturateOnIntegerOverflow=on  OutDataTypeStr=Inherit: Same as first input
  tc.plant.init.ratio : Gain  Gain=tc4.plant.init.ratio
  trq losses : Subsystem  mask(Lookup Table (2-D)){x=tc4.plant.init.trq_loss.idx1_trq, y=tc4.plant.init.trq_loss.idx2_spd, t=tc4.plant.init.trq_loss.map}
      mask prompts: x "Row:"; y "Column:"; t "Table:"
      mask help: Performs 2-D linear interpolation of input values using the specified input/output table. Extrapolation is performed outside the table boundaries.
      mask init:
      | [r,c]=size(t);
      | xt=reshape(x,prod(size(x)),1);
      | xi=xt(:,ones(1,c));
      | minx=min(x); maxx=max(x);
      | mint=min(min(t)); maxt=max(max(t));
      mask Display: plot(xi,t,[minx maxx],[mint mint],[minx minx],[mint maxt])
  trq out : Outport
  wires:
  Abs/1 -> trq losses/1(Rows)
  Abs1/1 -> trq losses/2(Cols)
  trq losses/1(Out1) -> Blending (state dependent)/1(Input)
  Blending (state dependent)/1(Output) -> Sum2/2
  spd in/1 -> Abs1/1, Blending (state dependent)/2(Control (state))
  trq in/1 -> Abs/1, Sum2/1
  Sum2/1 -> tc.plant.init.ratio/1
  tc.plant.init.ratio/1 -> trq out/1

== system AeroPropRefFranc/Propulsion and Aerodynamic Forces and Moments/S-Function/Battery Model/ess (battery)/ctrl/ess_ctrl_pngv_map_anl_PI_cstr/PI controller for maximal charge power and current1/PI Ratio Calculator (curr) /non-zero division1 ==
  note: and finally, the expression is: (u[1] \ u[2]) * 1 = u[1] \ u[2]
  note: (u[2]!=0) is true then returns 1
  note: if u[2] != 0, then output == u[1]\u[2]:
  note: (u[2]==0) is false then returns 0, thus (u[2]+(u[2]==0)) is equal to u[2]+0=u[2]
  note: and finally, the expression is: (u[1] \ 1) * 0 = 0
  note: (u[2]!=0) is false then returns 0
  note: if u[2] == 0, then output == 0:
  note: (u[2]==0) is true then returns 1, thus (u[2]+(u[2]==0)) is equal to 0+1=1
  note: original idea from Phil Sharer - ANL
      | original formula: u[1]\(u[2]+eps)*(u[2]!=0)
      | changes done by Gerald ZINI (dgey) - ANL (05\02\2001)
  In1 : Inport
  In2 : Inport  Port=2
  Fcn : Fcn  Expr=u[1]/(u[2]+(u[2]==0))*(u[2]!=0)
  Mux : Mux  Inputs=2
  Out1 : Outport
  wires:
  In2/1 -> Mux/2
  Fcn/1 -> Out1/1
  In1/1 -> Mux/1
  Mux/1 -> Fcn/1

== system AeroPropRefFranc/Propulsion and Aerodynamic Forces and Moments/S-Function/Battery Model/ess (battery)/ctrl/ess_ctrl_pngv_map_anl_PI_cstr/PI controller for maximal charge power and current1/PI Ratio Calculator (curr) 1/non-zero division1 ==
  note: and finally, the expression is: (u[1] \ u[2]) * 1 = u[1] \ u[2]
  note: (u[2]!=0) is true then returns 1
  note: if u[2] != 0, then output == u[1]\u[2]:
  note: (u[2]==0) is false then returns 0, thus (u[2]+(u[2]==0)) is equal to u[2]+0=u[2]
  note: and finally, the expression is: (u[1] \ 1) * 0 = 0
  note: (u[2]!=0) is false then returns 0
  note: if u[2] == 0, then output == 0:
  note: (u[2]==0) is true then returns 1, thus (u[2]+(u[2]==0)) is equal to 0+1=1
  note: original idea from Phil Sharer - ANL
      | original formula: u[1]\(u[2]+eps)*(u[2]!=0)
      | changes done by Gerald ZINI (dgey) - ANL (05\02\2001)
  In1 : Inport
  In2 : Inport  Port=2
  Fcn : Fcn  Expr=u[1]/(u[2]+(u[2]==0))*(u[2]!=0)
  Mux : Mux  Inputs=2
  Out1 : Outport
  wires:
  In2/1 -> Mux/2
  Fcn/1 -> Out1/1
  In1/1 -> Mux/1
  Mux/1 -> Fcn/1

== system AeroPropRefFranc/Propulsion and Aerodynamic Forces and Moments/S-Function/Battery Model/ess (battery)/ctrl/ess_ctrl_pngv_map_anl_PI_cstr/PI controller for maximal discharge power and current1/PI Ratio Calculator (curr) /non-zero division1 ==
  note: original idea from Phil Sharer - ANL
      | original formula: u[1]\(u[2]+eps)*(u[2]!=0)
      | changes done by Gerald ZINI (dgey) - ANL (05\02\2001)
  note: (u[2]==0) is true then returns 1, thus (u[2]+(u[2]==0)) is equal to 0+1=1
  note: if u[2] == 0, then output == 0:
  note: (u[2]!=0) is false then returns 0
  note: and finally, the expression is: (u[1] \ 1) * 0 = 0
  note: (u[2]==0) is false then returns 0, thus (u[2]+(u[2]==0)) is equal to u[2]+0=u[2]
  note: if u[2] != 0, then output == u[1]\u[2]:
  note: (u[2]!=0) is true then returns 1
  note: and finally, the expression is: (u[1] \ u[2]) * 1 = u[1] \ u[2]
  In1 : Inport
  In2 : Inport  Port=2
  Fcn : Fcn  Expr=u[1]/(u[2]+(u[2]==0))*(u[2]!=0)
  Mux : Mux  Inputs=2
  Out1 : Outport
  wires:
  Mux/1 -> Fcn/1
  In1/1 -> Mux/1
  Fcn/1 -> Out1/1
  In2/1 -> Mux/2

== system AeroPropRefFranc/Propulsion and Aerodynamic Forces and Moments/S-Function/Battery Model/ess (battery)/ctrl/ess_ctrl_pngv_map_anl_PI_cstr/PI controller for maximal discharge power and current1/PI Ratio Calculator (curr) 1/non-zero division1 ==
  note: and finally, the expression is: (u[1] \ u[2]) * 1 = u[1] \ u[2]
  note: (u[2]!=0) is true then returns 1
  note: if u[2] != 0, then output == u[1]\u[2]:
  note: (u[2]==0) is false then returns 0, thus (u[2]+(u[2]==0)) is equal to u[2]+0=u[2]
  note: and finally, the expression is: (u[1] \ 1) * 0 = 0
  note: (u[2]!=0) is false then returns 0
  note: if u[2] == 0, then output == 0:
  note: (u[2]==0) is true then returns 1, thus (u[2]+(u[2]==0)) is equal to 0+1=1
  note: original idea from Phil Sharer - ANL
      | original formula: u[1]\(u[2]+eps)*(u[2]!=0)
      | changes done by Gerald ZINI (dgey) - ANL (05\02\2001)
  In1 : Inport
  In2 : Inport  Port=2
  Fcn : Fcn  Expr=u[1]/(u[2]+(u[2]==0))*(u[2]!=0)
  Mux : Mux  Inputs=2
  Out1 : Outport
  wires:
  In2/1 -> Mux/2
  Fcn/1 -> Out1/1
  In1/1 -> Mux/1
  Mux/1 -> Fcn/1

== system AeroPropRefFranc/Propulsion and Aerodynamic Forces and Moments/S-Function/Battery Model/powerplant/ess (battery)/ctrl/ess_ctrl_pngv_map_anl_PI_cstr/PI controller for maximal charge power and current1/PI Ratio Calculator (curr)  ==
  note: %deviation
  ess curr : Inport
  curr max cont : Inport  Port=2
  Add1 : Sum  Inputs=-+
  Integrator1 : Integrator  InitialCondition=ess.plant.init.ul_curr_chg  LimitOutput=on  UpperSaturationLimit=ess.plant.init.ul_curr_chg  LowerSaturationLimit=ess.plant.init.ll_curr_chg
  Ki_curr : Gain  Gain=ess.plant.init.Ki_curr_chg  SaturateOnIntegerOverflow=on  OutDataTypeStr=Inherit: Same as input  ParamDataTypeStr=Inherit: Same as input
  Saturation1 : Saturate  UpperLimit=1  LowerLimit=0
  non-zero division1 : Subsystem
      mask Display: disp('divider')
  Current ratio : Outport
  wires:
  curr max cont/1 -> non-zero division1/2(In2), Add1/2
  Saturation1/1 -> Current ratio/1
  ess curr/1 -> Add1/1
  Integrator1/1 -> Saturation1/1
  Ki_curr/1 -> Integrator1/1
  non-zero division1/1(Out1) -> Ki_curr/1
  Add1/1 -> non-zero division1/1(In1)

== system AeroPropRefFranc/Propulsion and Aerodynamic Forces and Moments/S-Function/Battery Model/powerplant/ess (battery)/ctrl/ess_ctrl_pngv_map_anl_PI_cstr/PI controller for maximal charge power and current1/PI Ratio Calculator (curr) 1 ==
  note: %deviation
  ess pwr : Inport
  pwr max cont : Inport  Port=2
  Add1 : Sum  Inputs=-+
  Integrator1 : Integrator  InitialCondition=ess.plant.init.ul_curr_dis  LimitOutput=on  UpperSaturationLimit=ess.plant.init.ul_curr_dis  LowerSaturationLimit=ess.plant.init.ll_curr_dis
  Ki_pwr : Gain  Gain=ess.plant.init.Ki_pwr_chg  SaturateOnIntegerOverflow=on  OutDataTypeStr=Inherit: Same as input  ParamDataTypeStr=Inherit: Same as input
  Saturation1 : Saturate  UpperLimit=1  LowerLimit=0
  non-zero division1 : Subsystem
      mask Display: disp('divider')
  pwr ratio : Outport
  wires:
  pwr max cont/1 -> non-zero division1/2(In2), Add1/2
  Saturation1/1 -> pwr ratio/1
  ess pwr/1 -> Add1/1
  Integrator1/1 -> Saturation1/1
  Ki_pwr/1 -> Integrator1/1
  non-zero division1/1(Out1) -> Ki_pwr/1
  Add1/1 -> non-zero division1/1(In1)

== system AeroPropRefFranc/Propulsion and Aerodynamic Forces and Moments/S-Function/Battery Model/powerplant/ess (battery)/ctrl/ess_ctrl_pngv_map_anl_PI_cstr/PI controller for maximal discharge power and current1/PI Ratio Calculator (curr)  ==
  note: %deviation
  ess curr : Inport
  curr max cont : Inport  Port=2
  Add1 : Sum  Inputs=-+
  Integrator1 : Integrator  InitialCondition=ess.plant.init.ul_curr_dis  LimitOutput=on  UpperSaturationLimit=ess.plant.init.ul_curr_dis  LowerSaturationLimit=ess.plant.init.ll_curr_dis
  Ki_curr : Gain  Gain=ess.plant.init.Ki_curr_dis  SaturateOnIntegerOverflow=on  OutDataTypeStr=Inherit: Same as input  ParamDataTypeStr=Inherit: Same as input
  Saturation1 : Saturate  UpperLimit=1  LowerLimit=0
  non-zero division1 : Subsystem
      mask Display: disp('divider')
  Current ratio : Outport
  wires:
  Add1/1 -> non-zero division1/1(In1)
  non-zero division1/1(Out1) -> Ki_curr/1
  Ki_curr/1 -> Integrator1/1
  Integrator1/1 -> Saturation1/1
  ess curr/1 -> Add1/1
  Saturation1/1 -> Current ratio/1
  curr max cont/1 -> Add1/2, non-zero division1/2(In2)

== system AeroPropRefFranc/Propulsion and Aerodynamic Forces and Moments/S-Function/Battery Model/powerplant/ess (battery)/ctrl/ess_ctrl_pngv_map_anl_PI_cstr/PI controller for maximal discharge power and current1/PI Ratio Calculator (curr) 1 ==
  note: %deviation
  ess pwr : Inport
  pwr max cont : Inport  Port=2
  Add1 : Sum  Inputs=-+
  Integrator1 : Integrator  InitialCondition=ess.plant.init.ul_curr_dis  LimitOutput=on  UpperSaturationLimit=ess.plant.init.ul_curr_dis  LowerSaturationLimit=ess.plant.init.ll_curr_dis
  Ki_pwr : Gain  Gain=ess.plant.init.Ki_pwr_dis  SaturateOnIntegerOverflow=on  OutDataTypeStr=Inherit: Same as input  ParamDataTypeStr=Inherit: Same as input
  Saturation1 : Saturate  UpperLimit=1  LowerLimit=0
  non-zero division1 : Subsystem
      mask Display: disp('divider')
  pwr ratio : Outport
  wires:
  pwr max cont/1 -> non-zero division1/2(In2), Add1/2
  Saturation1/1 -> pwr ratio/1
  ess pwr/1 -> Add1/1
  Integrator1/1 -> Saturation1/1
  Ki_pwr/1 -> Integrator1/1
  non-zero division1/1(Out1) -> Ki_pwr/1
  Add1/1 -> non-zero division1/1(In1)

== system AeroPropRefFranc/Propulsion and Aerodynamic Forces and Moments/S-Function/Battery Model/powerplant/ess (battery)/plant/ess_plant_pngv_map_anl_PI_cstr/ess_cell/current polarization ==
  ess soc : Inport
  ess curr : Inport  Port=2
  Integrator : Integrator
  Product1 : Product  Inputs=*/  InputSameDT=on  SaturateOnIntegerOverflow=on  OutDataTypeStr=Inherit: Same as first input
  Sum1 : Sum  Inputs=+-  InputSameDT=on  SaturateOnIntegerOverflow=on  OutDataTypeStr=Inherit: Same as first input
  Time Constant : Lookup  InputValues=ess.plant.init.tau1.idx1_soc  Table=ess.plant.init.tau1.map
  ess_cell_curr_polar1 : Outport
  wires:
  Integrator/1 -> ess_cell_curr_polar1/1, Sum1/2
  Sum1/1 -> Product1/1
  ess curr/1 -> Sum1/1
  ess soc/1 -> Time Constant/1
  Product1/1 -> Integrator/1
  Time Constant/1 -> Product1/2

== system AeroPropRefFranc/Propulsion and Aerodynamic Forces and Moments/S-Function/Battery Model/powerplant/ess (battery)/plant/ess_plant_pngv_map_anl_PI_cstr/ess_cell/current polarization1 ==
  ess soc : Inport
  ess curr : Inport  Port=2
  Integrator : Integrator
  Product1 : Product  Inputs=*/  InputSameDT=on  SaturateOnIntegerOverflow=on  OutDataTypeStr=Inherit: Same as first input
  Sum1 : Sum  Inputs=+-  InputSameDT=on  SaturateOnIntegerOverflow=on  OutDataTypeStr=Inherit: Same as first input
  Time Constant : Lookup  InputValues=ess.plant.init.tau2.idx1_soc  Table=ess.plant.init.tau2.map
  ess_cell_curr_polar2 : Outport
  wires:
  Time Constant/1 -> Product1/2
  Product1/1 -> Integrator/1
  ess soc/1 -> Time Constant/1
  ess curr/1 -> Sum1/1
  Sum1/1 -> Product1/1
  Integrator/1 -> Sum1/2, ess_cell_curr_polar2/1

== system AeroPropRefFranc/Propulsion and Aerodynamic Forces and Moments/S-Function/Battery Model/powerplant/ess (battery)/plant/ess_plant_pngv_map_anl_PI_cstr/ess_cell/ess_soc_calculation ==
  cell_curr : Inport
  (sec->hrs) : Gain  Gain=1/3600  SaturateOnIntegerOverflow=on  OutDataTypeStr=Inherit: Same as input  ParamDataTypeStr=Inherit: Same as input
  (sec->hrs)1 : Gain  Gain=-1  SaturateOnIntegerOverflow=on  OutDataTypeStr=Inherit: Same as input  ParamDataTypeStr=Inherit: Same as input
  0 <= SOC <= 1 : Saturate  UpperLimit=1  LowerLimit=0
  1\ess.plant.init.cap : Gain  Gain=1/ess.plant.init.cap  SaturateOnIntegerOverflow=on  OutDataTypeStr=Inherit: Same as input  ParamDataTypeStr=Inherit: Same as input
  Integrator : Integrator  InitialCondition=ess.plant.init.soc_init
  ess_soc : Outport
  wires:
  cell_curr/1 -> (sec->hrs)/1
  1\ess.plant.init.cap/1 -> (sec->hrs)1/1
  (sec->hrs)1/1 -> Integrator/1
  Integrator/1 -> 0 <= SOC <= 1/1
  0 <= SOC <= 1/1 -> ess_soc/1
  (sec->hrs)/1 -> 1\ess.plant.init.cap/1

== system AeroPropRefFranc/Propulsion and Aerodynamic Forces and Moments/S-Function/Battery Model/powerplant/ess (battery)/plant/ess_plant_pngv_map_anl_PI_cstr/ess_cell/voltage calculation ==
  absolute SOC : Inport
  ess_cell_curr : Inport  Port=2
  ess_cell_curr_pol1 : Inport  Port=3
  ess_cell_curr_plo2 : Inport  Port=4
  Ohmic resist : Lookup  InputValues=ess.plant.init.rint.idx1_soc  Table=ess.plant.init.rint.map
  "Polarization resist 2 " : Lookup  InputValues=ess.plant.init.rpol2.idx1_soc  Table=ess.plant.init.rpol2.map
  Polarization resist2 : Lookup  InputValues=ess.plant.init.rpol1.idx1_soc  Table=ess.plant.init.rpol1.map
  Product1 : Product  InputSameDT=on  SaturateOnIntegerOverflow=on  OutDataTypeStr=Inherit: Same as first input
  Product2 : Product  InputSameDT=on  SaturateOnIntegerOverflow=on  OutDataTypeStr=Inherit: Same as first input
  Product3 : Product  InputSameDT=on  SaturateOnIntegerOverflow=on  OutDataTypeStr=Inherit: Same as first input
  Saturation : Saturate  UpperLimit=inf  LowerLimit=ess.plant.init.volt_min_burst
  Sum2 : Sum  Inputs=+---  InputSameDT=on  SaturateOnIntegerOverflow=on  OutDataTypeStr=Inherit: Same as first input
  Voc : Lookup  InputValues=ess.plant.init.voc.idx1_soc  Table=ess.plant.init.voc.map
  ess_cell_volt : Outport
  ess_cell_voc : Outport  Port=2
  ess_cell_rint : Outport  Port=3
  ess_cell_rpol1 : Outport  Port=4
  ess_cell_rpol2 : Outport  Port=5
  wires:
  Sum2/1 -> Saturation/1
  Ohmic resist/1 -> Product1/2, ess_cell_rint/1  "ess_rint_simu"
  ess_cell_curr/1 -> Product1/1
  Voc/1 -> Sum2/1, ess_cell_voc/1  "ess_voc_simu"
  absolute SOC/1 -> Voc/1, Ohmic resist/1, "Polarization resist 2 "/1, Polarization resist2/1
  Product1/1 -> Sum2/2
  ess_cell_curr_pol1/1 -> Product2/1
  Polarization resist2/1 -> Product2/2, ess_cell_rpol1/1  "ess_rpol1_simu"
  Product2/1 -> Sum2/3
  Product3/1 -> Sum2/4
  ess_cell_curr_plo2/1 -> Product3/1
  "Polarization resist 2 "/1 -> Product3/2, ess_cell_rpol2/1  "ess_rpol2_simu"
  Saturation/1 -> ess_cell_volt/1

== system AeroPropRefFranc/Propulsion and Aerodynamic Forces and Moments/S-Function/Battery Model/powerplant/ess (battery)1/ctrl/ess_ctrl_pngv_map_anl_PI_cstr/PI controller for maximal charge power and current1/PI Ratio Calculator (curr)  ==
  note: %deviation
  ess curr : Inport
  curr max cont : Inport  Port=2
  Add1 : Sum  Inputs=-+
  Integrator1 : Integrator  InitialCondition=ess.plant.init.ul_curr_chg  LimitOutput=on  UpperSaturationLimit=ess.plant.init.ul_curr_chg  LowerSaturationLimit=ess.plant.init.ll_curr_chg
  Ki_curr : Gain  Gain=ess.plant.init.Ki_curr_chg  SaturateOnIntegerOverflow=on  OutDataTypeStr=Inherit: Same as input  ParamDataTypeStr=Inherit: Same as input
  Saturation1 : Saturate  UpperLimit=1  LowerLimit=0
  non-zero division1 : Subsystem
      mask Display: disp('divider')
  Current ratio : Outport
  wires:
  Add1/1 -> non-zero division1/1(In1)
  non-zero division1/1(Out1) -> Ki_curr/1
  Ki_curr/1 -> Integrator1/1
  Integrator1/1 -> Saturation1/1
  ess curr/1 -> Add1/1
  Saturation1/1 -> Current ratio/1
  curr max cont/1 -> Add1/2, non-zero division1/2(In2)
